simulink model "MatLab4"  (Simulink 8.7)
settings: Solver=ode45  StartTime=0.0  StopTime=8  MaxStep=0.01  RelTol=1e-3
values from neighbouring files (symbols this model uses):
  A = [0 1  0              0 ... (first row only)    [MatLab4p.m]    (also in MatLab5p.m = [     0        1       0        0; MatLab6p_solucao4.m = [     0        1       0        0; MatLab7p.m = [0 1; -5*sqrt(2) -1]; pplane8.m = [)
  B = [0; 1/M; 0; -1/(M*L)]    [MatLab4p.m]    (also in MatLab5p.m = [ 0    0; MatLab6p_solucao4.m = [ 0    0; MatLab7p.m = [0 ; 10]; pplane8.m = real(A))
  C = [1 0 0 0]    [MatLab4p.m]    (also in MatLab5p.m = [1 0 0 0; MatLab6p_solucao4.m = [1 0 0 0; MatLab7p.m = [1 0]; pplane8.m = imag(A))
  Dsim = zeros(4,1)    [MatLab4p.m]    (also in MatLab5p.m = zeros(4,2); MatLab6p_solucao4.m = zeros(4,2); questao2Miguel.m; questao2MiguelFinal.m)
  K = place(A,B,[-3 -3.05 -3.1 -3.15])    [MatLab4p.m]    (also in MatLab5p.m = Ka(:,1:4); MatLab6p_solucao4.m = Ka(:,1:4); MatLab7p.m = place(A,B,[-4 -4.05]); pplane8.m = kk +2*(jj-1))
  L = (place(A',C',[-9 -9.05 -9.1 -9.15]))'    [MatLab4p.m]    (also in MatLab7p.m = [23 ; 113.9289]; PenduloInvertidoNLinear.m = 1; pplane8.m = length(t); questao2Miguel.m = 1)
  x0 = [0 0 pi/4 0]    [MatLab4p.m]    (also in MatLab5p.m = [1 0.5 1 0.1]; MatLab6p_solucao4.m = [0 0 0 0]; MatLab7p.m = [0 ; 0]; questao2Miguel.m = [0 0.01 0.3 0])
  x0obs = [0 0 0 0]    [MatLab4p.m]    (also in MatLab6p_solucao4.m; MatLab7p.m = [0 ; 0]; questao2Miguel.m; questao2MiguelFinal.m)
settings Model: Creator=hector  LastModifiedBy=Deinis-UFSC
settings DebuggingCC: UnderspecifiedInitializationDetection=Simplified  MergeDetectMultiDrivingBlocksExec=error  SolverPrmCheckMsg=warning
settings ConfigComp: CovSFcnEnable=off

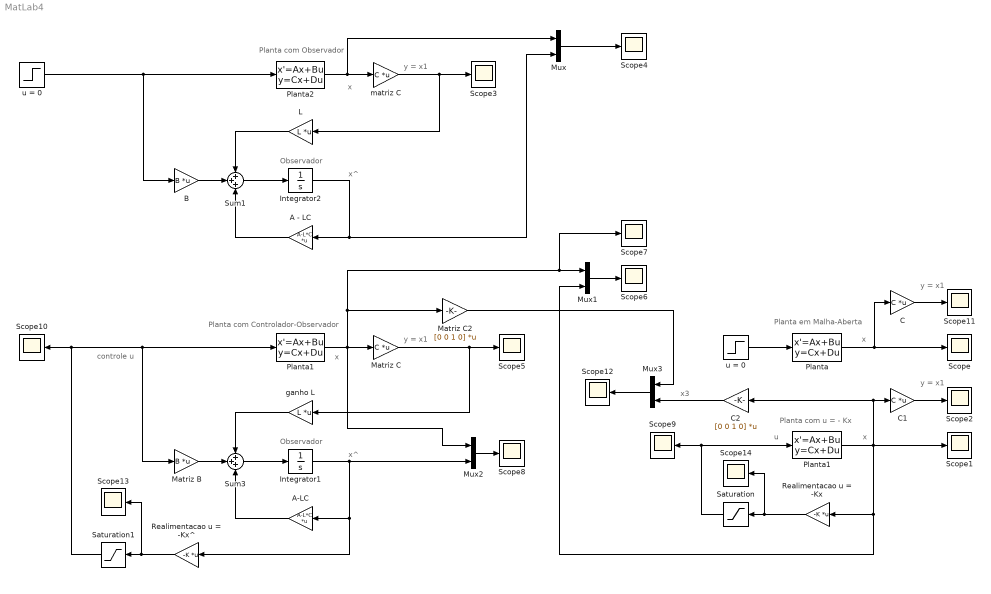
== system MatLab4 ==
  note: x3
  note: x
  note: controle u
  note: Observador
  note: Planta com Controlador-Observador
  note: Observador
  note: Planta com Observador
  note: Planta com u = - Kx
  note: Planta em Malha-Aberta
  note: x^
  note: x
  note: x^
  note: x
  note: u
  note: x
  note: y = x1
  note: y = x1
  note: y = x1
  note: y = x1
  "       Realimentacao u = -Kx^" : Gain  Gain=-K  Multiplication=Matrix(K*u)
  A - LC : Gain  Gain=A-L*C  Multiplication=Matrix(K*u)
  A-LC : Gain  Gain=A-L*C  Multiplication=Matrix(K*u)
  B : Gain  Gain=B  Multiplication=Matrix(K*u)
  C : Gain  Gain=C  Multiplication=Matrix(K*u)
  C1 : Gain  Gain=C  Multiplication=Matrix(K*u)
  C2 : Gain  Gain=[0 0 1 0]  Multiplication=Matrix(K*u)
  Integrator1 : Integrator  InitialCondition=x0obs
  Integrator2 : Integrator  InitialCondition=x0obs
  L : Gain  Gain=L  Multiplication=Matrix(K*u)
  Matriz B : Gain  Gain=B  Multiplication=Matrix(K*u)
  "Matriz C " : Gain  Gain=C  Multiplication=Matrix(K*u)
  Matriz C2 : Gain  Gain=[0 0 1 0]  Multiplication=Matrix(K*u)
  Mux{,1..3} (4 alike) : Mux  Inputs=2
  Planta : StateSpace  A=A  B=B  C=eye(4)  D=Dsim  X0=x0
  Planta1 : StateSpace  A=A  B=B  C=eye(4)  D=Dsim  X0=x0
  "Planta1 " : StateSpace  A=A  B=B  C=eye(4)  D=Dsim  X0=x0
  Planta2 : StateSpace  A=A  B=B  C=eye(4)  D=Dsim  X0=x0
  Realimentacao u = -Kx : Gain  Gain=-K  Multiplication=Matrix(K*u)
  Saturation : Saturate  UpperLimit=40  LowerLimit=-40
  Saturation1 : Saturate  UpperLimit=40  LowerLimit=-40
  Scope{,1..14} (15 alike) : Scope
  Sum1 : Sum  Inputs=+++
  Sum3 : Sum  Inputs=+++
  ganho L : Gain  Gain=L  Multiplication=Matrix(K*u)
  matriz C : Gain  Gain=C  Multiplication=Matrix(K*u)
  u = 0 : Step  Time=0  After=0  SampleTime=0
  "u = 0 " : Step  Time=0  After=0  SampleTime=0
  wires:
  u = 0/1 -> Planta/1
  Realimentacao u = -Kx/1 -> Scope14/1, Saturation/1
  "Planta1 "/1 -> Scope1/1, Mux1/2, Realimentacao u = -Kx/1, C2/1, C1/1
  C1/1 -> Scope2/1
  "u = 0 "/1 -> Planta2/1, B/1
  Planta2/1 -> Mux/1, matriz C/1
  Integrator2/1 -> Mux/2, A - LC/1
  matriz C/1 -> L/1, Scope3/1
  L/1 -> Sum1/1
  Sum1/1 -> Integrator2/1
  A - LC/1 -> Sum1/3
  B/1 -> Sum1/2
  Mux/1 -> Scope4/1
  "       Realimentacao u = -Kx^"/1 -> Scope13/1, Saturation1/1
  Integrator1/1 -> "       Realimentacao u = -Kx^"/1, A-LC/1, Mux2/2
  "Matriz C "/1 -> ganho L/1, Scope5/1
  ganho L/1 -> Sum3/1
  Sum3/1 -> Integrator1/1
  Mux1/1 -> Scope6/1
  Planta1/1 -> "Matriz C "/1, Mux2/1, Scope7/1, Mux1/1, Matriz C2/1
  Mux2/1 -> Scope8/1
  A-LC/1 -> Sum3/3
  Matriz B/1 -> Sum3/2
  Planta/1 -> C/1, Scope/1
  C/1 -> Scope11/1
  Saturation/1 -> "Planta1 "/1, Scope9/1
  Saturation1/1 -> Planta1/1, Matriz B/1, Scope10/1
  Matriz C2/1 -> Mux3/1
  C2/1 -> Mux3/2
  Mux3/1 -> Scope12/1
